simulink model "Junctions1"  (Simulink 5.0)
settings: Solver=ode45  StartTime=0.0  StopTime=10.0  RelTol=1e-3
settings Model: Creator=scaife  LastModifiedBy=scaife  ExtModeAutoUpdateStatusClock=off

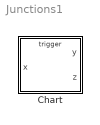
== system Junctions1 ==
  Chart : Stateflow chart

== stateflow chart Chart ==
  state A
  state B
  state C
  (default) -> A
  A -> (junction 6) : E1[x>0]{y++}/z+=2
  (junction 6) -> C : [x<=2]{y++}/z++
  (junction 6) -> B : [x>2]{y+=2}/z++;z++
  C -> A : [x>3]
  B -> A : [x>3]
  data: x input int32; y output int32 =1; z output int32 =2
  events: E1 input EITHER_EDGE_EVENT
